simulink model "TessOneMotor"  (R2021b)
settings: Solver=ode8  StartTime=0.0  StopTime=3  FixedStep=200e-6  MaxStep=1e-4  RelTol=1e-3  EnableMultiTasking=on
values from neighbouring files (symbols this model uses):
  bEMFConstant = 0.0081    [DC_Motor_InitParam.m]
  Den_b = 2*Damp*Wn    (= 56.5486677646)    [DC_Motor_InitParam.m]
  Den_c = Wn^2    (= 986.960440109)    [DC_Motor_InitParam.m]
  Inductance = Resistance*Te    (= 0.00157625)    [DC_Motor_InitParam.m]
  Inertia = 9.89e-06    [DC_Motor_InitParam.m]
  Num = Wn^2*Gain    (= 1947948.23706)    [DC_Motor_InitParam.m]
  Resistance = 3.25    [DC_Motor_InitParam.m]
  TorqueConstant = bEMFConstant    (= 0.0081)    [DC_Motor_InitParam.m]
libraries: simulink x2, slpidlib x1
settings Model: Creator=IulVas  LastModifiedBy=axinteandrei
settings SolverCC: AlgebraicLoopSolver=TrustRegion
settings DataIOCC: LimitDataPoints=on  SaveFormat=Array  SignalLoggingSaveFormat=ModelDataLogs  ReturnWorkspaceOutputs=off  SignalLoggingName=sigsOut
settings OptimizationCC: BooleanDataType=off  InitFltsAndDblsToZero=on  LifeSpan=inf
settings DebuggingCC: SaveWithParameterizedLinksMsg=none  UnderspecifiedInitializationDetection=Classic  MergeDetectMultiDrivingBlocksExec=none  SignalResolutionControl=TryResolveAllWithWarning  MultiTaskDSMMsg=warning  MultiTaskCondExecSysMsg=none  FcnCallInpInsideContextMsg=warning  SFUnexpectedBacktrackingDiag=warning  SFNoUnconditionalDefaultTransitionDiag=warning  SFMachineParentedDataDiag=warning  ArithmeticOperatorsInVariantConditions=warning
settings HardwareCC: ProdBitPerPointer=32  ProdBitPerSizeT=32  ProdBitPerPtrDiffT=32  ProdLargestAtomicFloat=None  ProdIntDivRoundTo=Undefined  ProdEndianess=Unspecified  ProdWordSize=32  ProdHWDeviceType=32-bit Generic  TargetUnknown=on
settings ModelReferenceCC: PropagateSignalLabelsOutOfModel=off
settings SFSimCC: SimUseLocalCustomCode=off  CustomCodeUndefinedFunction=UseInterfaceOnly
settings RTWCC: RTWUseLocalCustomCode=off
settings CodeAppCC: StateflowObjectComments=on
settings GRTTargetCC: TargetLangStandard=C89/C90 (ANSI)  CombineOutputUpdateFcns=off  GRTInterface=on
settings ConfigComp: CovMetricSettings=dw  CovSaveCumulativeToWorkspaceVar=on  CovSaveSingleToWorkspaceVar=on  CovExternalEMLEnable=off

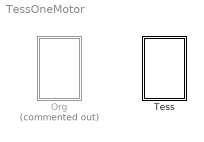
== system TessOneMotor ==
  Org : Subsystem  Commented=on
  Tess : Subsystem

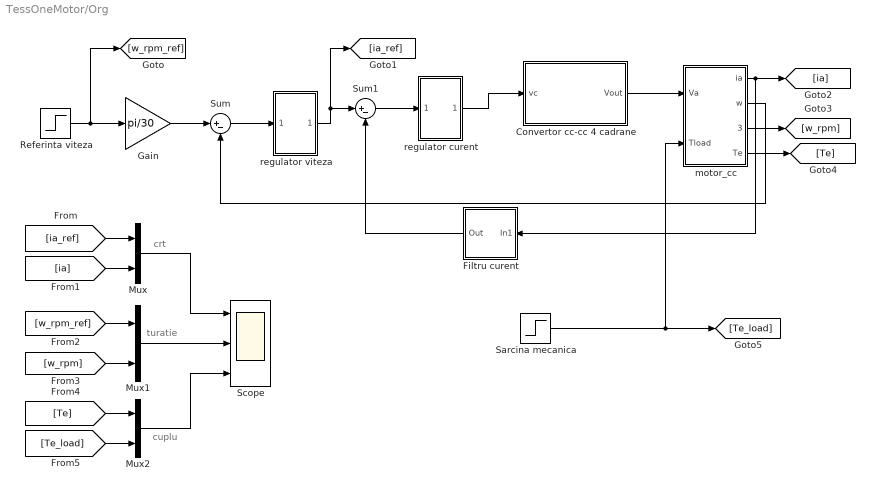
== system TessOneMotor/Org ==
  note: crt
  note: turatie
  note: cuplu
  Convertor cc-cc 4 cadrane : Subsystem  mask{Vd=200, fsw=10}
      mask prompts: Vd "Supply Voltage Vd (V)"; fsw "Switching frequency (kHz)"
  Filtru curent : Subsystem  mask{fc=5000}
      mask prompts: fc "Frecventa taiere [Hz]"
      mask init:
      | Tf=1/(2*pi*fc);
  Gain : Gain  Gain=pi/30  SaturateOnIntegerOverflow=on  OutDataTypeStr=Inherit: Same as input  ParamDataTypeStr=Inherit: Same as input
  Mux : Mux  Inputs=2
  Mux1 : Mux  Inputs=2
  Mux2 : Mux  Inputs=2
  Referinta viteza : Step  Time=0.2  Before=-2000  After=2000  SampleTime=0
  Sarcina mecanica : Step  Time=0.35  After=10  SampleTime=0
  Scope : Scope  NumInputPorts=3
  Sum : Sum  Inputs=|+-  SaturateOnIntegerOverflow=on
  Sum1 : Sum  Inputs=|+-  SaturateOnIntegerOverflow=on
  motor_cc : Subsystem  mask{Vd=200, Tload=10, Ra=0.37, La=1.5e-3, k_T=0.5, k_E=0.5, D=0, J=0.008}
      mask prompts: Vd "Tensiune alimentare [V]"; Tload "Cuplu sarcina"; Ra "Rezistenta indusului [ohm]"; La "Inductanta indusului [H]"; k_T "Constanta cuplului [Nm/A]"; k_E "Constanta tensiunii electromecanice [V/(rad/sec)]"; D "Coeficient de frecare vascoasa [Nm/(rad/sec)]"; J "Moment de inertie total [kgm^2]"
  regulator curent : Subsystem  mask{ki=2.32, kp=0.94e-2}
  "regulator viteza " : Subsystem  mask{ki=126.08, kp=1.74}
  wires:
  Referinta viteza/1 -> Gain/1, [w_rpm_ref]
  [ia_ref] -> Mux/1
  "regulator viteza "/1(com) -> [ia_ref], Sum1/1
  Sarcina mecanica/1 -> [Te_load], motor_cc/2(Tload)
  regulator curent/1(com) -> Convertor cc-cc 4 cadrane/1(vc)
  [Te] -> Mux2/1
  Mux1/1 -> Scope/2
  Mux2/1 -> Scope/3
  Sum/1 -> "regulator viteza "/1(error)
  motor_cc/1(ia) -> [ia], Filtru curent/1(In1)
  Filtru curent/1(Out) -> Sum1/2
  motor_cc/4(Te) -> [Te]
  [Te_load] -> Mux2/2
  Mux/1 -> Scope/1
  [ia] -> Mux/2
  Gain/1 -> Sum/1
  [w_rpm_ref] -> Mux1/1
  [w_rpm] -> Mux1/2
  Sum1/1 -> regulator curent/1(error)
  Convertor cc-cc 4 cadrane/1(Vout) -> motor_cc/1(Va)
  motor_cc/2(w) -> Sum/2
  motor_cc/3(w_rpm) -> [w_rpm]

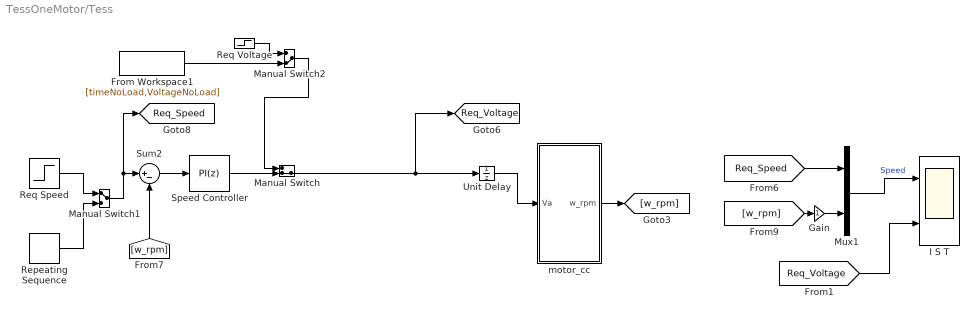
== system TessOneMotor/Tess ==
  From Workspace1 : FromWorkspace  VariableName=[timeNoLoad,VoltageNoLoad]  SampleTime=-1
  Gain : Gain
  I S T : Scope  NumInputPorts=2
  Manual Switch : ManualSwitch  CurrentSetting=0
  Manual Switch1 : ManualSwitch
  Manual Switch2 : ManualSwitch  CurrentSetting=0
  Mux1 : Mux  Inputs=2
  Repeating Sequence : simulink/Sources/Repeating Sequence  rep_seq_t=[0 0.5 1 1.5 2 2.5 ]  rep_seq_y=[0 2000 0 10000 -10000 0]
  Req Speed : Step  Time=0.05  After=7500
  Req Voltage : Step  Time=0.05  After=4
  Speed Controller : slpidlib/PID Controller  Controller=PI  Form=Parallel  TimeDomain=Discrete-time  UseExternalTs=off  SampleTime=-1  IntegratorMethod=Forward Euler  FilterMethod=Forward Euler  ControllerParametersSource=internal  P=0.229398906164868  I=2.68049691525518  D=0  UseFilter=on  N=100  TunerSelectOption=Transfer Function Based (PID Tuner App)  InitialConditionSource=internal  InitialConditionForIntegrator=0  InitialConditionForFilter=0  DifferentiatorICPrevScaledInput=0  ExternalReset=none  TrackingMode=off  Kt=1  LimitOutput=on  SatLimitsSource=internal  UpperSaturationLimit=4.5  LowerSaturationLimit=-4.5  LinearizeAsGain=on  AntiWindupMode=clamping  Kb=0.3  POutMin=[]  POutMax=[]  IOutMin=[]  IOutMax=[]  DOutMin=[]  DOutMax=[]  NOutMin=[]  NOutMax=[]  SumOutMin=[]  SumOutMax=[]  SaturationOutMin=[]  SaturationOutMax=[]  PParamMin=[]  PParamMax=[]  IParamMin=[]  IParamMax=[]  DParamMin=[]  DParamMax=[]  NParamMin=[]  NParamMax=[]  KbParamMin=[]  KbParamMax=[]  KtParamMin=[]  KtParamMax=[]  KbOutMin=[]  KbOutMax=[]  KtOutMin=[]  KtOutMax=[]  IntegratorOutMin=[]  IntegratorOutMax=[]  FilterOutMin=[]  FilterOutMax=[]  SumI1OutMin=[]  SumI1OutMax=[]  SumI2OutMin=[]  SumI2OutMax=[]  SumI3OutMin=[]  SumI3OutMax=[]  SumI4OutMin=[]  SumI4OutMax=[]  SumDOutMin=[]  SumDOutMax=[]  DifferentiatorOutMin=[]  DifferentiatorOutMax=[]  FilterDiffOutCoefMin=[]  FilterDiffOutCoefMax=[]  ReciprocalOutMin=[]  ReciprocalOutMax=[]  SumDenOutMin=[]  SumDenOutMax=[]  SumNumOutMin=[]  SumNumOutMax=[]  DivideOutMin=[]  DivideOutMax=[]  UdiffTsProdOutMin=[]  UdiffTsProdOutMax=[]  NTsProdOutMin=[]  NTsProdOutMax=[]  UintegralTsProdOutMin=[]  UintegralTsProdOutMax=[]  UngainTsProdOutMin=[]  UngainTsProdOutMax=[]  IntegratorContinuousStateAttributes=''  IntegratorStateMustResolveToSignalObject=off  IntegratorRTWStateStorageClass=Auto  FilterContinuousStateAttributes=''  FilterStateMustResolveToSignalObject=off  FilterRTWStateStorageClass=Auto  ParallelPVariant=InternalParameters  IdealPVariant=Disabled  IVariant=InternalParameters  DVariant=Disabled  IntegratorVariant=Discrete  SatVariant=Enabled  AWVariant=DiscClampingParallel  PCopyVariant=Disabled  TRVariant=Disabled  FdbkBlocksVariant=Forward  IdealPFdbkVariant=Disabled  SatFdbkVariant=Disabled  DerivativeFilterVariant=Disabled  NVariant=Disabled  NCopyVariant=Disabled_SignalSpec  FilterICVariant=Disabled  IntegratorICVariant=InternalICs  ExternalResetVariant=Disabled  TRSumVariant=Passthrough  SumFdbkVariant=Disabled  SumVariant=Sum_PI  TsampFilterVariant=InternalTs  TsampNgainVariant=Passthrough  TsampIntegralVariant=Passthrough  ExternalSaturationOutDataTypeStr=Inherit: Same as second input
  Sum2 : Sum  Inputs=|+-  SaturateOnIntegerOverflow=on
  Unit Delay : UnitDelay  SampleTime=-1  HasFrameUpgradeWarning=on
  motor_cc : Subsystem  mask{Vd=5.1, Tload=0, Ra=2, La=651e-6, k_T=0.0035, k_E=0.0035, D=0, J=0.00000028}
      mask prompts: Vd "Tensiune alimentare [V]"; Tload "Cuplu sarcina"; Ra "Rezistenta indusului [ohm]"; La "Inductanta indusului [H]"; k_T "Constanta cuplului [Nm/A]"; k_E "Constanta tensiunii electromecanice [V/(rad/sec)]"; D "Coeficient de frecare vascoasa [Nm/(rad/sec)]"; J "Moment de inertie total [kgm^2]"
  tag scope: Req_Speed=global, Req_Voltage=global
  wires:
  motor_cc/1(w_rpm) -> [w_rpm]
  Mux1/1 -> I S T/1  "Speed"
  Sum2/1 -> Speed Controller/1
  [Req_Speed] -> Mux1/1
  [w_rpm] -> Gain/1
  Gain/1 -> Mux1/2
  [w_rpm] -> Sum2/2
  Unit Delay/1 -> motor_cc/1(Va)
  Manual Switch/1 -> [Req_Voltage], Unit Delay/1
  Speed Controller/1 -> Manual Switch/2
  Manual Switch1/1 -> [Req_Speed], Sum2/1
  Req Speed/1 -> Manual Switch1/1
  Repeating Sequence/1 -> Manual Switch1/2
  Req Voltage/1 -> Manual Switch2/1
  Manual Switch2/1 -> Manual Switch/1
  From Workspace1/1 -> Manual Switch2/2
  [Req_Voltage] -> I S T/2

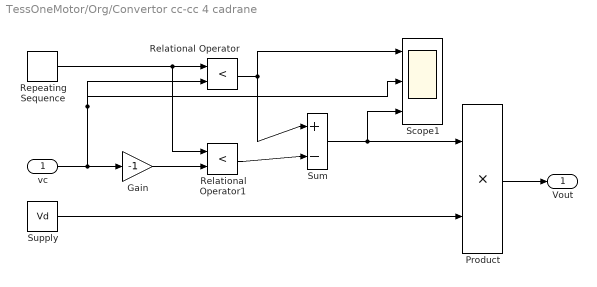
== system TessOneMotor/Org/Convertor cc-cc 4 cadrane ==
  vc : Inport
  Gain : Gain  Gain=-1  SaturateOnIntegerOverflow=on  OutDataTypeStr=Inherit: Same as input  ParamDataTypeStr=Inherit: Same as input
  Product : Product  SaturateOnIntegerOverflow=on  OutDataTypeStr=Inherit: Same as first input
  Relational Operator : RelationalOperator  Operator=<  RndMeth=Nearest
  Relational Operator1 : RelationalOperator  Operator=<  RndMeth=Nearest
  Repeating Sequence : simulink/Sources/Repeating Sequence  rep_seq_t=[0 0.5e-3/10 1e-3/10]  rep_seq_y=[-1 1 -1]
  Scope1 : Scope  NumInputPorts=3
  Sum : Sum  Inputs=|+-  SaturateOnIntegerOverflow=on
  Supply : Constant  Value=Vd
  Vout : Outport
  wires:
  Supply/1 -> Product/2
  Gain/1 -> Relational Operator1/2
  vc/1 -> Gain/1, Relational Operator/2, Scope1/2
  Repeating Sequence/1 -> Relational Operator1/1, Relational Operator/1
  Product/1 -> Vout/1
  Sum/1 -> Product/1, Scope1/3
  Relational Operator1/1 -> Sum/2
  Relational Operator/1 -> Sum/1, Scope1/1

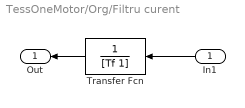
== system TessOneMotor/Org/Filtru curent ==
  In1 : Inport
  Transfer Fcn : TransferFcn  Denominator=[Tf 1]
  Out : Outport
  wires:
  In1/1 -> Transfer Fcn/1
  Transfer Fcn/1 -> Out/1

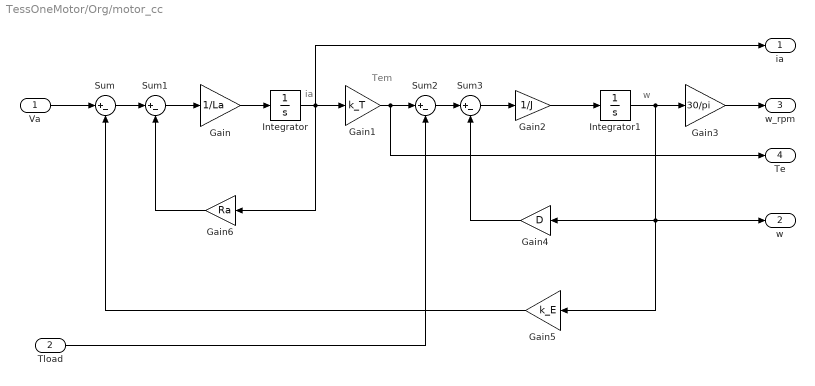
== system TessOneMotor/Org/motor_cc ==
  note: w
  note: Tem
  note: ia
  Va : Inport
  Tload : Inport  Port=2
  Gain : Gain  Gain=1/La  SaturateOnIntegerOverflow=on  OutDataTypeStr=Inherit: Same as input  ParamDataTypeStr=Inherit: Same as input
  Gain1 : Gain  Gain=k_T  SaturateOnIntegerOverflow=on  OutDataTypeStr=Inherit: Same as input  ParamDataTypeStr=Inherit: Same as input
  Gain2 : Gain  Gain=1/J  SaturateOnIntegerOverflow=on  OutDataTypeStr=Inherit: Same as input  ParamDataTypeStr=Inherit: Same as input
  Gain3 : Gain  Gain=30/pi  SaturateOnIntegerOverflow=on  OutDataTypeStr=Inherit: Same as input  ParamDataTypeStr=Inherit: Same as input
  Gain4 : Gain  Gain=D  SaturateOnIntegerOverflow=on  OutDataTypeStr=Inherit: Same as input  ParamDataTypeStr=Inherit: Same as input
  Gain5 : Gain  Gain=k_E  SaturateOnIntegerOverflow=on  OutDataTypeStr=Inherit: Same as input  ParamDataTypeStr=Inherit: Same as input
  Gain6 : Gain  Gain=Ra  SaturateOnIntegerOverflow=on  OutDataTypeStr=Inherit: Same as input  ParamDataTypeStr=Inherit: Same as input
  Integrator : Integrator
  Integrator1 : Integrator
  Sum{,1..3} (4 alike) : Sum  Inputs=|+-  SaturateOnIntegerOverflow=on
  ia : Outport
  w : Outport  Port=2
  w_rpm : Outport  Port=3
  Te : Outport  Port=4
  wires:
  Gain4/1 -> Sum3/2
  Gain6/1 -> Sum1/2
  Gain5/1 -> Sum/2
  Integrator1/1 -> Gain3/1, w/1, Gain4/1, Gain5/1
  Gain2/1 -> Integrator1/1
  Sum3/1 -> Gain2/1
  Sum2/1 -> Sum3/1
  Gain1/1 -> Te/1, Sum2/1
  Integrator/1 -> ia/1, Gain6/1, Gain1/1
  Gain/1 -> Integrator/1
  Sum1/1 -> Gain/1
  Sum/1 -> Sum1/1
  Gain3/1 -> w_rpm/1
  Va/1 -> Sum/1
  Tload/1 -> Sum2/2

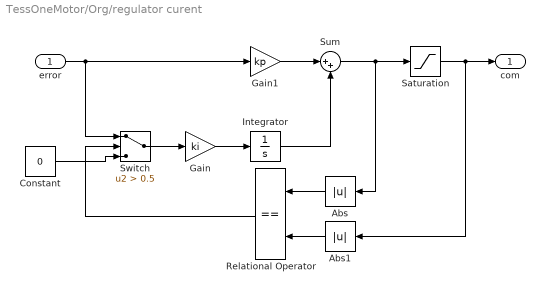
== system TessOneMotor/Org/regulator curent ==
  error : Inport
  Abs : Abs  SaturateOnIntegerOverflow=on
  Abs1 : Abs  SaturateOnIntegerOverflow=on
  Constant : Constant  Value=0
  Gain : Gain  Gain=ki  SaturateOnIntegerOverflow=on  OutDataTypeStr=Inherit: Same as input  ParamDataTypeStr=Inherit: Same as input
  Gain1 : Gain  Gain=kp  SaturateOnIntegerOverflow=on  OutDataTypeStr=Inherit: Same as input  ParamDataTypeStr=Inherit: Same as input
  Integrator : Integrator
  Relational Operator : RelationalOperator  Operator===  RndMeth=Nearest
  Saturation : Saturate  UpperLimit=1  LowerLimit=-1
  Sum : Sum  Inputs=|++  SaturateOnIntegerOverflow=on
  Switch : Switch  Criteria=u2 > Threshold  Threshold=0.5
  com : Outport
  wires:
  error/1 -> Gain1/1, Switch/1
  Switch/1 -> Gain/1
  Gain/1 -> Integrator/1
  Integrator/1 -> Sum/2
  Gain1/1 -> Sum/1
  Sum/1 -> Saturation/1, Abs/1
  Saturation/1 -> com/1, Abs1/1
  Abs/1 -> Relational Operator/1
  Abs1/1 -> Relational Operator/2
  Relational Operator/1 -> Switch/2
  Constant/1 -> Switch/3

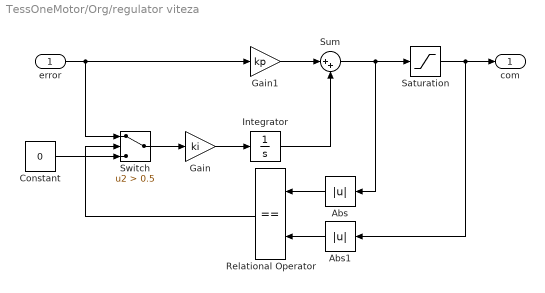
== system TessOneMotor/Org/regulator viteza  ==
  error : Inport
  Abs : Abs  SaturateOnIntegerOverflow=on
  Abs1 : Abs  SaturateOnIntegerOverflow=on
  Constant : Constant  Value=0
  Gain : Gain  Gain=ki  SaturateOnIntegerOverflow=on  OutDataTypeStr=Inherit: Same as input  ParamDataTypeStr=Inherit: Same as input
  Gain1 : Gain  Gain=kp  SaturateOnIntegerOverflow=on  OutDataTypeStr=Inherit: Same as input  ParamDataTypeStr=Inherit: Same as input
  Integrator : Integrator
  Relational Operator : RelationalOperator  Operator===  RndMeth=Nearest
  Saturation : Saturate  UpperLimit=50  LowerLimit=-50
  Sum : Sum  Inputs=|++  SaturateOnIntegerOverflow=on
  Switch : Switch  Criteria=u2 > Threshold  Threshold=0.5
  com : Outport
  wires:
  Constant/1 -> Switch/3
  Relational Operator/1 -> Switch/2
  Abs1/1 -> Relational Operator/2
  Abs/1 -> Relational Operator/1
  Saturation/1 -> Abs1/1, com/1
  Sum/1 -> Abs/1, Saturation/1
  Gain1/1 -> Sum/1
  Integrator/1 -> Sum/2
  Gain/1 -> Integrator/1
  Switch/1 -> Gain/1
  error/1 -> Switch/1, Gain1/1

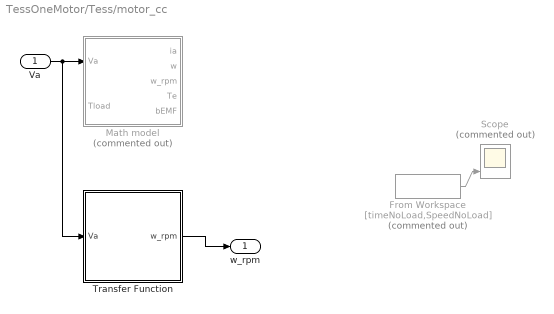
== system TessOneMotor/Tess/motor_cc ==
  Va : Inport
  From Workspace : FromWorkspace  Commented=on  VariableName=[timeNoLoad,SpeedNoLoad]  SampleTime=-1
  Math model : Subsystem  Commented=on
  Scope : Scope  Commented=on  NumInputPorts=3
  Transfer Function : Subsystem
  w_rpm : Outport
  wires:
  Va/1 -> Transfer Function/1(Va), Math model/1(Va)
  From Workspace/1 -> Scope/3
  Transfer Function/1(w_rpm) -> w_rpm/1

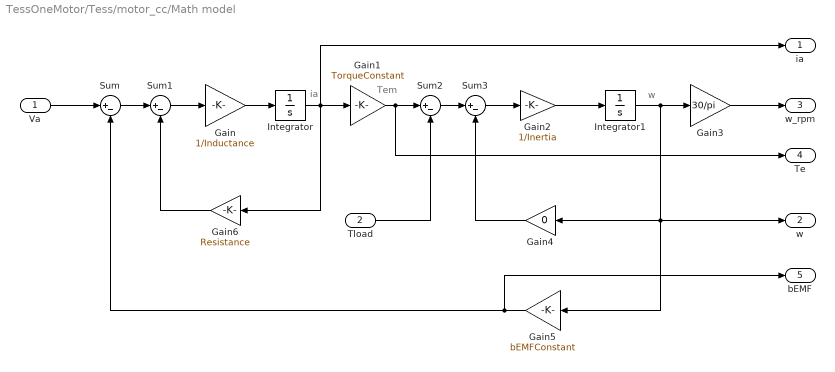
== system TessOneMotor/Tess/motor_cc/Math model ==
  note: w
  note: Tem
  note: ia
  Va : Inport
  Tload : Inport  Port=2
  Gain : Gain  Gain=1/Inductance  SaturateOnIntegerOverflow=on  OutDataTypeStr=Inherit: Same as input  ParamDataTypeStr=Inherit: Same as input
  Gain1 : Gain  Gain=TorqueConstant  SaturateOnIntegerOverflow=on  OutDataTypeStr=Inherit: Same as input  ParamDataTypeStr=Inherit: Same as input
  Gain2 : Gain  Gain=1/Inertia  SaturateOnIntegerOverflow=on  OutDataTypeStr=Inherit: Same as input  ParamDataTypeStr=Inherit: Same as input
  Gain3 : Gain  Gain=30/pi  SaturateOnIntegerOverflow=on  OutDataTypeStr=Inherit: Same as input  ParamDataTypeStr=Inherit: Same as input
  Gain4 : Gain  Gain=0  SaturateOnIntegerOverflow=on  OutDataTypeStr=Inherit: Same as input  ParamDataTypeStr=Inherit: Same as input
  Gain5 : Gain  Gain=bEMFConstant  SaturateOnIntegerOverflow=on  OutDataTypeStr=Inherit: Same as input  ParamDataTypeStr=Inherit: Same as input
  Gain6 : Gain  Gain=Resistance  SaturateOnIntegerOverflow=on  OutDataTypeStr=Inherit: Same as input  ParamDataTypeStr=Inherit: Same as input
  Integrator : Integrator
  Integrator1 : Integrator
  Sum{,1..3} (4 alike) : Sum  Inputs=|+-  SaturateOnIntegerOverflow=on
  ia : Outport
  w : Outport  Port=2
  w_rpm : Outport  Port=3
  Te : Outport  Port=4
  bEMF : Outport  Port=5
  wires:
  Gain1/1 -> Te/1, Sum2/1
  Sum2/1 -> Sum3/1
  Va/1 -> Sum/1
  Sum1/1 -> Gain/1
  Gain2/1 -> Integrator1/1
  Integrator1/1 -> Gain3/1, w/1, Gain4/1, Gain5/1
  Sum3/1 -> Gain2/1
  Sum/1 -> Sum1/1
  Tload/1 -> Sum2/2
  Gain4/1 -> Sum3/2
  Integrator/1 -> ia/1, Gain6/1, Gain1/1
  Gain6/1 -> Sum1/2
  Gain3/1 -> w_rpm/1
  Gain/1 -> Integrator/1
  Gain5/1 -> bEMF/1, Sum/2

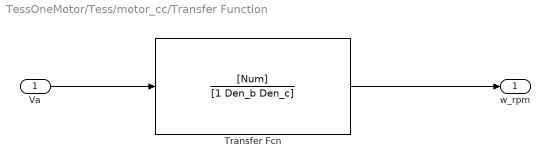
== system TessOneMotor/Tess/motor_cc/Transfer Function ==
  Va : Inport
  Transfer Fcn : TransferFcn  Numerator=[Num]  Denominator=[1 Den_b Den_c]
  w_rpm : Outport
  wires:
  Transfer Fcn/1 -> w_rpm/1
  Va/1 -> Transfer Fcn/1
